simulink model "model2_raw"  (Simulink 7.7)
settings: Solver=VariableStepDiscrete  StartTime=0.0  StopTime=kk  RelTol=1e-3
values from neighbouring files (symbols this model uses):
  A = A1'    [dyskretny.m]    (also in przebieg.m; zmiennestanu.m)
  B = C1'    [dyskretny.m]    (also in przebieg.m; zmiennestanu.m)
libraries: simulink x3
settings Model: Creator=Andones  LastModifiedBy=qiubix

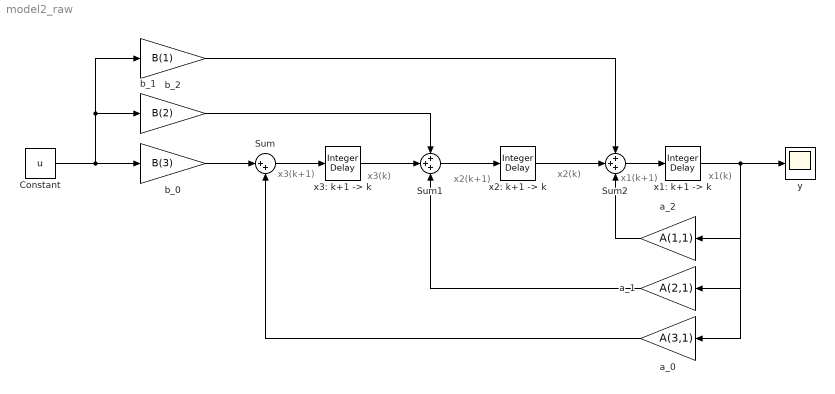
== system model2_raw ==
  note: x3(k+1)
  note: x3(k)
  note: x2(k+1)
  note: x2(k)
  note: x1(k+1)
  note: x1(k)
  " x1: k+1 -> k" : simulink/Discrete/Integer Delay  NumDelays=1  vinit=1  samptime=T_s
  Constant : Constant  Value=u
  Sum : Sum  Inputs=|++
  Sum1 : Sum  Inputs=+++
  Sum2 : Sum  Inputs=+++
  a_0 : Gain  Gain=A(3,1)
  a_1 : Gain  Gain=A(2,1)
  a_2 : Gain  Gain=A(1,1)
  b_0 : Gain  Gain=B(3)
  b_1 : Gain  Gain=B(2)
  b_2 : Gain  Gain=B(1)
  "x2: k+1 -> k" : simulink/Discrete/Integer Delay  NumDelays=1  vinit=-1  samptime=T_s
  "x3: k+1 -> k " : simulink/Discrete/Integer Delay  NumDelays=1  vinit=-1  samptime=T_s
  y : Scope
  wires:
  Sum2/1 -> " x1: k+1 -> k"/1
  " x1: k+1 -> k"/1 -> y/1, a_2/1, a_1/1, a_0/1
  Sum/1 -> "x3: k+1 -> k "/1
  "x3: k+1 -> k "/1 -> Sum1/2
  Sum1/1 -> "x2: k+1 -> k"/1
  a_2/1 -> Sum2/3
  a_1/1 -> Sum1/3
  b_1/1 -> Sum1/1
  b_2/1 -> Sum2/1
  b_0/1 -> Sum/1
  a_0/1 -> Sum/2
  "x2: k+1 -> k"/1 -> Sum2/2
  Constant/1 -> b_0/1, b_1/1, b_2/1
